simulink model "sesto"  (R2023a)
settings: Solver=VariableStepAuto  StartTime=0.0  StopTime=20/((2*pi)/w)  MaxStep=((2*pi)/w)/1000  RelTol=1e-3
model workspace (MAT data in the model file):
  R = 0.5
  XC = -1
  XL1 = 1
  XL2 = 2
  XM = 1
  w = 6.28318530718
libraries: fl_lib x21, nesl_utility x4
settings Model: Creator=Aguer  LastModifiedBy=Aguer

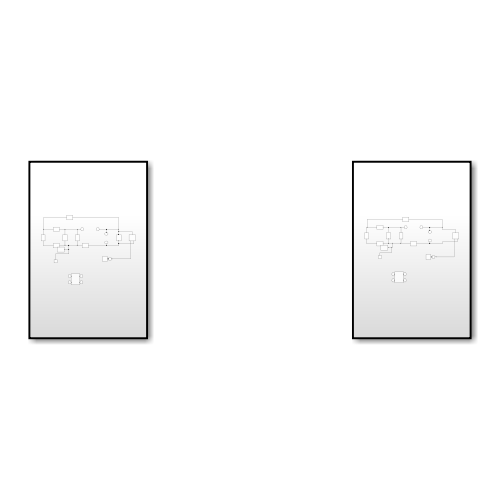
[thumbnail: Simulink's stored preview of the top-level diagram]
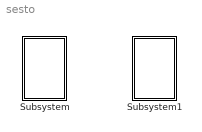
== system sesto ==
  Subsystem : Subsystem
  Subsystem1 : Subsystem

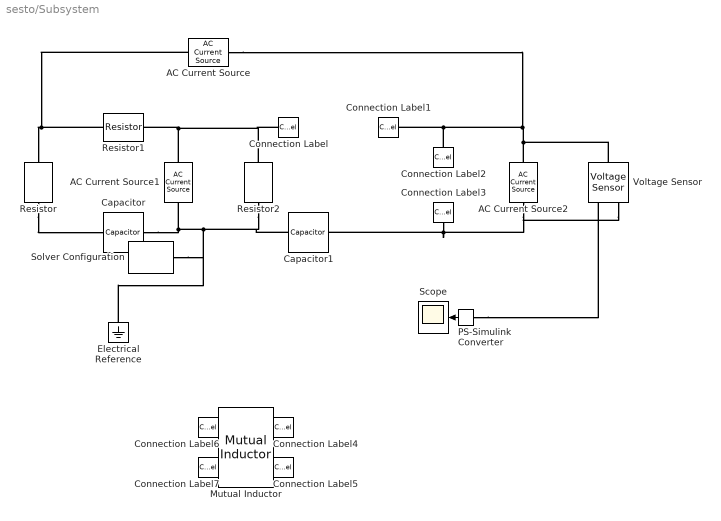
== system sesto/Subsystem ==
  AC Current Source : fl_lib/Electrical/Electrical Sources/AC Current Source  amp=0 A  shift=90 deg  frequency=w/(2*pi) Hz  omega=0 rad/s
      settings: InternalSimscapePortConfiguration="{\"Bottom\":[],\"Left\":[{\"id\":\"p\",\"label\":\"\",\"type\":\"foundation.electrical.electrical\"}],\"Right\":[{\"id\":\"n\",\"label\":\"\",\"type\":\"foundation.electrical.electrical\"}],\"Top\":[]}"
  AC Current Source1 : fl_lib/Electrical/Electrical Sources/AC Current Source  amp=0 A  shift=90 deg  frequency=w/(2*pi) Hz  omega=0 rad/s
      settings: InternalSimscapePortConfiguration="{\"Bottom\":[],\"Left\":[{\"id\":\"p\",\"label\":\"\",\"type\":\"foundation.electrical.electrical\"}],\"Right\":[{\"id\":\"n\",\"label\":\"\",\"type\":\"foundation.electrical.electrical\"}],\"Top\":[]}"
  AC Current Source2 : fl_lib/Electrical/Electrical Sources/AC Current Source  amp=1 A  shift=90 deg  frequency=w/(2*pi) Hz  omega=0 rad/s
      settings: InternalSimscapePortConfiguration="{\"Bottom\":[],\"Left\":[{\"id\":\"p\",\"label\":\"\",\"type\":\"foundation.electrical.electrical\"}],\"Right\":[{\"id\":\"n\",\"label\":\"\",\"type\":\"foundation.electrical.electrical\"}],\"Top\":[]}"
  Capacitor : fl_lib/Electrical/Electrical Elements/Capacitor  c=-1/(w*XC) F  r=0 Ohm  g=0 1/Ohm  i_specify=off  i_priority=None  i=0 A  i_nominal_specify=off  i_nominal_unit=A  i_nominal_value=1  v_specify=off  v_priority=None  v=0 V  v_nominal_specify=off  v_nominal_unit=V  v_nominal_value=1  vc_specify=off  vc_priority=High  vc=0 V  vc_nominal_specify=off  vc_nominal_unit=V  vc_nominal_value=1
  Capacitor1 : fl_lib/Electrical/Electrical Elements/Capacitor  c=-1/(w*XC) F  r=0 Ohm  g=0 1/Ohm  i_specify=off  i_priority=None  i=0 A  i_nominal_specify=off  i_nominal_unit=A  i_nominal_value=1  v_specify=off  v_priority=None  v=0 V  v_nominal_specify=off  v_nominal_unit=V  v_nominal_value=1  vc_specify=off  vc_priority=High  vc=0 V  vc_nominal_specify=off  vc_nominal_unit=V  vc_nominal_value=1
  Connection Label : ConnectionLabel  Label=ind_n1
  Connection Label1 : ConnectionLabel  Label=ind_p1
  Connection Label2 : ConnectionLabel  Label=ind_p2
  Connection Label3 : ConnectionLabel  Label=ind_n2
  Connection Label4 : ConnectionLabel  Label=ind_p2
  Connection Label5 : ConnectionLabel  Label=ind_n2
  Connection Label6 : ConnectionLabel  Label=ind_p1
  Connection Label7 : ConnectionLabel  Label=ind_n1
  Electrical Reference : fl_lib/Electrical/Electrical Elements/Electrical Reference
  Mutual Inductor : fl_lib/Electrical/Electrical Elements/Mutual Inductor  L1=XL1/w H  L2=XL2/w H  k=XM/(sqrt(XL1*XL2))  i1_specify=off  i1_priority=High  i1=0 A  i1_nominal_specify=off  i1_nominal_unit=A  i1_nominal_value=1  i2_specify=off  i2_priority=High  i2=0 A  i2_nominal_specify=off  i2_nominal_unit=A  i2_nominal_value=1  v1_specify=off  v1_priority=None  v1=0 V  v1_nominal_specify=off  v1_nominal_unit=V  v1_nominal_value=1  v2_specify=off  v2_priority=None  v2=0 V  v2_nominal_specify=off  v2_nominal_unit=V  v2_nominal_value=1
      settings: InternalSimscapePortConfiguration="{\"Bottom\":[],\"Left\":[{\"id\":\"p1\",\"label\":\"1+\",\"type\":\"foundation.electrical.electrical\"},{\"id\":\"n1\",\"label\":\"1-\",\"type\":\"foundation.electrical.electrical\"}],\"Right\":[{\"id\":\"p2\",\"label\":\"2+\",\"type\":\"foundation.electrical.electrical\"},{\"id\":\"n2\",\"label\":\"2-\",\"type\":\"foundation.electrical.electrical\"}],\"Top\":[]}"
  PS-Simulink Converter : nesl_utility/PS-Simulink Converter  PhysicalDomain=network_engine_domain  SubClassName=ps_output  LeftPortType=input  RightPortType=output  PseudoPeriodic=off  Frequencies=[]  VectorFormat=inherit  Unit=inherit  AffineConversion=off
  Resistor : fl_lib/Electrical/Electrical Elements/Resistor  R=R Ohm  i_specify=off  i_priority=None  i=0 A  i_nominal_specify=off  i_nominal_unit=A  i_nominal_value=1  v_specify=off  v_priority=None  v=0 V  v_nominal_specify=off  v_nominal_unit=V  v_nominal_value=1
  Resistor1 : fl_lib/Electrical/Electrical Elements/Resistor  R=R Ohm  i_specify=off  i_priority=None  i=0 A  i_nominal_specify=off  i_nominal_unit=A  i_nominal_value=1  v_specify=off  v_priority=None  v=0 V  v_nominal_specify=off  v_nominal_unit=V  v_nominal_value=1
  Resistor2 : fl_lib/Electrical/Electrical Elements/Resistor  R=R Ohm  i_specify=off  i_priority=None  i=0 A  i_nominal_specify=off  i_nominal_unit=A  i_nominal_value=1  v_specify=off  v_priority=None  v=0 V  v_nominal_specify=off  v_nominal_unit=V  v_nominal_value=1
  Scope : Scope
  Solver Configuration : nesl_utility/Solver Configuration  PhysicalDomain=network_engine_domain  SubClassName=solver  LeftPortType=input  RightPortType=generic  Tones=[]  Harmonics=[]  SimulateNoise=off  Profile=off  UseLocalSampling=off  EnableSwitchedLinearOptims=on  FrequencyDomain=off  UseCCode=off  RelTol=0.001  AbsTol=0.001  MinStep=1e-09  ToWorkspace=off  RevertToSquareIcSolve=off  NumHomotopyIterations=100  PhasorMode=off  PhasorModeNumHarmonics=1  ConsistencySolver=NEWTON_XTOL_AFTER_FTOL  IndexReductionMethod=DerivativeReplacement  DoDC=off  ResidualTolerance=1e-09  ConsistencyTolSource=GLOBAL  ConsistencyAbsTol=0.001  ConsistencyRelTol=0.001  ConsistencyTolFactor=0.001  UseLocalSolver=off  LocalSolverChoice=NE_BACKWARD_EULER_ADVANCER  ResolveIndetEquations=on  FunctionEvalNumThread=1  LocalSolverSampleTime=0.001  DoFixedCost=off  MaxNonlinIter=3  MaxModeIter=2  ComputeImpulses=off  ImpulseIterations=2  LinearAlgebra=auto  LinearAlgebraNumThread=0  EquationFormulation=NE_TIME_EF  DelaysMemoryBudget=1024  AutomaticFiltering=on  FilteringTimeConstant=0.001  PartitionStorageMethod=AS_NEEDED  PartitionMemoryBudget=1024  PartitionMethod=ROBUST
  Voltage Sensor : fl_lib/Electrical/Electrical Sensors/Voltage Sensor
  wires:
  PS-Simulink Converter/1 -> Scope/1
  connections:
  Connection Label3/LConn1 -- Voltage Sensor/RConn2 -- AC Current Source2/RConn1 -- Capacitor1/RConn1
  Resistor1/LConn1 -- AC Current Source/RConn1 -- Resistor/LConn1
  Resistor/RConn1 -- Capacitor/LConn1
  AC Current Source2/LConn1 -- Voltage Sensor/LConn1 -- Connection Label1/LConn1 -- Connection Label2/LConn1 -- AC Current Source/LConn1
  AC Current Source1/LConn1 -- Connection Label/LConn1 -- Resistor2/LConn1 -- Resistor1/RConn1
  Capacitor/RConn1 -- Solver Configuration/RConn1 -- Electrical Reference/LConn1 -- Capacitor1/LConn1 -- Resistor2/RConn1 -- AC Current Source1/RConn1
  Connection Label5/LConn1 -- Mutual Inductor/RConn2
  Connection Label4/LConn1 -- Mutual Inductor/RConn1
  PS-Simulink Converter/LConn1 -- Voltage Sensor/RConn1
  Connection Label6/LConn1 -- Mutual Inductor/LConn1
  Connection Label7/LConn1 -- Mutual Inductor/LConn2

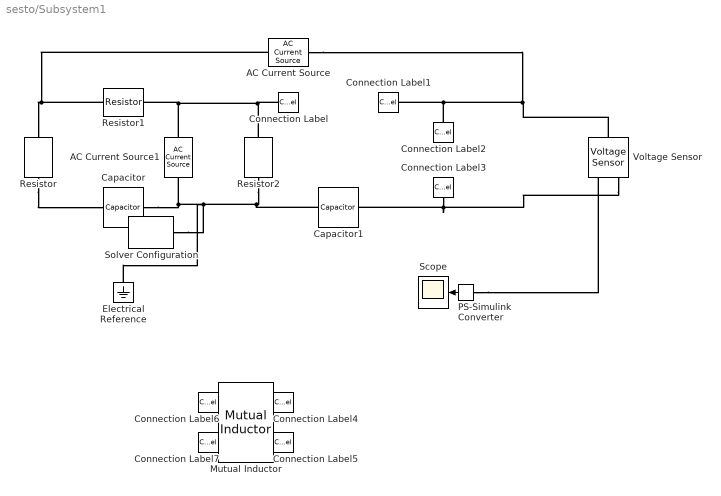
== system sesto/Subsystem1 ==
  AC Current Source : fl_lib/Electrical/Electrical Sources/AC Current Source  amp=4 A  shift=pi+(pi/2) rad  frequency=w/(2*pi) Hz  omega=0 rad/s
      settings: InternalSimscapePortConfiguration="{\"Bottom\":[],\"Left\":[{\"id\":\"p\",\"label\":\"\",\"type\":\"foundation.electrical.electrical\"}],\"Right\":[{\"id\":\"n\",\"label\":\"\",\"type\":\"foundation.electrical.electrical\"}],\"Top\":[]}"
  AC Current Source1 : fl_lib/Electrical/Electrical Sources/AC Current Source  amp=sqrt(2) A  shift=-(pi/4)+(pi/2) rad  frequency=w/(2*pi) Hz  omega=0 rad/s
      settings: InternalSimscapePortConfiguration="{\"Bottom\":[],\"Left\":[{\"id\":\"p\",\"label\":\"\",\"type\":\"foundation.electrical.electrical\"}],\"Right\":[{\"id\":\"n\",\"label\":\"\",\"type\":\"foundation.electrical.electrical\"}],\"Top\":[]}"
  Capacitor : fl_lib/Electrical/Electrical Elements/Capacitor  c=-1/(w*XC) F  r=0 Ohm  g=0 1/Ohm  i_specify=off  i_priority=None  i=0 A  i_nominal_specify=off  i_nominal_unit=A  i_nominal_value=1  v_specify=off  v_priority=None  v=0 V  v_nominal_specify=off  v_nominal_unit=V  v_nominal_value=1  vc_specify=off  vc_priority=High  vc=0 V  vc_nominal_specify=off  vc_nominal_unit=V  vc_nominal_value=1
  Capacitor1 : fl_lib/Electrical/Electrical Elements/Capacitor  c=-1/(w*XC) F  r=0 Ohm  g=0 1/Ohm  i_specify=off  i_priority=None  i=0 A  i_nominal_specify=off  i_nominal_unit=A  i_nominal_value=1  v_specify=off  v_priority=None  v=0 V  v_nominal_specify=off  v_nominal_unit=V  v_nominal_value=1  vc_specify=off  vc_priority=High  vc=0 V  vc_nominal_specify=off  vc_nominal_unit=V  vc_nominal_value=1
  Connection Label : ConnectionLabel  Label=ind_n1
  Connection Label1 : ConnectionLabel  Label=ind_p1
  Connection Label2 : ConnectionLabel  Label=ind_p2
  Connection Label3 : ConnectionLabel  Label=ind_n2
  Connection Label4 : ConnectionLabel  Label=ind_p2
  Connection Label5 : ConnectionLabel  Label=ind_n2
  Connection Label6 : ConnectionLabel  Label=ind_p1
  Connection Label7 : ConnectionLabel  Label=ind_n1
  Electrical Reference : fl_lib/Electrical/Electrical Elements/Electrical Reference
  Mutual Inductor : fl_lib/Electrical/Electrical Elements/Mutual Inductor  L1=XL1/w H  L2=XL2/w H  k=XM/(sqrt(XL1*XL2))  i1_specify=off  i1_priority=High  i1=0 A  i1_nominal_specify=off  i1_nominal_unit=A  i1_nominal_value=1  i2_specify=off  i2_priority=High  i2=0 A  i2_nominal_specify=off  i2_nominal_unit=A  i2_nominal_value=1  v1_specify=off  v1_priority=None  v1=0 V  v1_nominal_specify=off  v1_nominal_unit=V  v1_nominal_value=1  v2_specify=off  v2_priority=None  v2=0 V  v2_nominal_specify=off  v2_nominal_unit=V  v2_nominal_value=1
      settings: InternalSimscapePortConfiguration="{\"Bottom\":[],\"Left\":[{\"id\":\"p1\",\"label\":\"1+\",\"type\":\"foundation.electrical.electrical\"},{\"id\":\"n1\",\"label\":\"1-\",\"type\":\"foundation.electrical.electrical\"}],\"Right\":[{\"id\":\"p2\",\"label\":\"2+\",\"type\":\"foundation.electrical.electrical\"},{\"id\":\"n2\",\"label\":\"2-\",\"type\":\"foundation.electrical.electrical\"}],\"Top\":[]}"
  PS-Simulink Converter : nesl_utility/PS-Simulink Converter  PhysicalDomain=network_engine_domain  SubClassName=ps_output  LeftPortType=input  RightPortType=output  PseudoPeriodic=off  Frequencies=[]  VectorFormat=inherit  Unit=inherit  AffineConversion=off
  Resistor : fl_lib/Electrical/Electrical Elements/Resistor  R=R Ohm  i_specify=off  i_priority=None  i=0 A  i_nominal_specify=off  i_nominal_unit=A  i_nominal_value=1  v_specify=off  v_priority=None  v=0 V  v_nominal_specify=off  v_nominal_unit=V  v_nominal_value=1
  Resistor1 : fl_lib/Electrical/Electrical Elements/Resistor  R=R Ohm  i_specify=off  i_priority=None  i=0 A  i_nominal_specify=off  i_nominal_unit=A  i_nominal_value=1  v_specify=off  v_priority=None  v=0 V  v_nominal_specify=off  v_nominal_unit=V  v_nominal_value=1
  Resistor2 : fl_lib/Electrical/Electrical Elements/Resistor  R=R Ohm  i_specify=off  i_priority=None  i=0 A  i_nominal_specify=off  i_nominal_unit=A  i_nominal_value=1  v_specify=off  v_priority=None  v=0 V  v_nominal_specify=off  v_nominal_unit=V  v_nominal_value=1
  Scope : Scope
  Solver Configuration : nesl_utility/Solver Configuration  PhysicalDomain=network_engine_domain  SubClassName=solver  LeftPortType=input  RightPortType=generic  Tones=[]  Harmonics=[]  SimulateNoise=off  Profile=off  UseLocalSampling=off  EnableSwitchedLinearOptims=on  FrequencyDomain=off  UseCCode=off  RelTol=0.001  AbsTol=0.001  MinStep=1e-09  ToWorkspace=off  RevertToSquareIcSolve=off  NumHomotopyIterations=100  PhasorMode=off  PhasorModeNumHarmonics=1  ConsistencySolver=NEWTON_XTOL_AFTER_FTOL  IndexReductionMethod=DerivativeReplacement  DoDC=off  ResidualTolerance=1e-09  ConsistencyTolSource=GLOBAL  ConsistencyAbsTol=0.001  ConsistencyRelTol=0.001  ConsistencyTolFactor=0.001  UseLocalSolver=off  LocalSolverChoice=NE_BACKWARD_EULER_ADVANCER  ResolveIndetEquations=on  FunctionEvalNumThread=1  LocalSolverSampleTime=0.001  DoFixedCost=off  MaxNonlinIter=3  MaxModeIter=2  ComputeImpulses=off  ImpulseIterations=2  LinearAlgebra=auto  LinearAlgebraNumThread=0  EquationFormulation=NE_TIME_EF  DelaysMemoryBudget=1024  AutomaticFiltering=on  FilteringTimeConstant=0.001  PartitionStorageMethod=AS_NEEDED  PartitionMemoryBudget=1024  PartitionMethod=ROBUST
  Voltage Sensor : fl_lib/Electrical/Electrical Sensors/Voltage Sensor
  wires:
  PS-Simulink Converter/1 -> Scope/1
  connections:
  Connection Label4/LConn1 -- Mutual Inductor/RConn1
  Resistor1/LConn1 -- AC Current Source/RConn1 -- Resistor/LConn1
  Connection Label6/LConn1 -- Mutual Inductor/LConn1
  Resistor2/RConn1 -- Capacitor1/LConn1 -- Solver Configuration/RConn1 -- Electrical Reference/LConn1 -- AC Current Source1/RConn1 -- Capacitor/RConn1
  AC Current Source/LConn1 -- Voltage Sensor/LConn1 -- Connection Label1/LConn1 -- Connection Label2/LConn1
  Connection Label3/LConn1 -- Voltage Sensor/RConn2 -- Capacitor1/RConn1
  Resistor/RConn1 -- Capacitor/LConn1
  PS-Simulink Converter/LConn1 -- Voltage Sensor/RConn1
  Connection Label7/LConn1 -- Mutual Inductor/LConn2
  Resistor2/LConn1 -- Connection Label/LConn1 -- Resistor1/RConn1 -- AC Current Source1/LConn1
  Connection Label5/LConn1 -- Mutual Inductor/RConn2
